simulink model "Modello_corretto_1dof"  (R2023b)
settings: Solver=VariableStepAuto  StartTime=0.0  StopTime=100  RelTol=1e-3
undefined symbols (not defined in the file or in its folder): param, tau_eq, Ts_slk, x0
settings Model: Creator=asus  LastModifiedBy=asus
settings OptimizationCC: ReuseModelBlockBuffer=off
settings DebuggingCC: SignalInfNanChecking=error

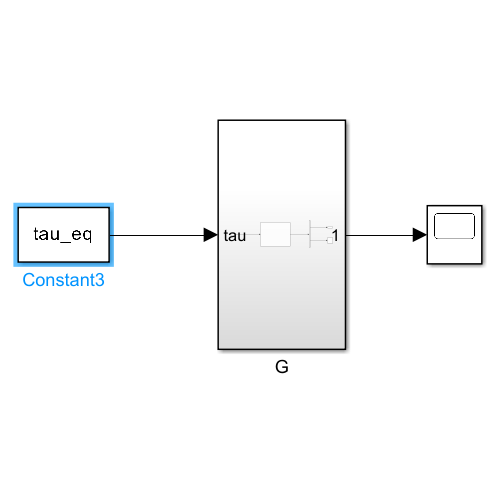
[thumbnail: Simulink's stored preview of the top-level diagram]
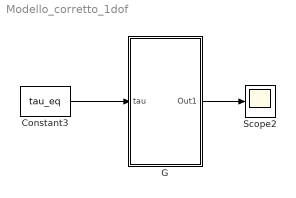
== system Modello_corretto_1dof ==
  Constant3 : Constant  Value=tau_eq  VectorParams1D=off  SampleTime=Ts_slk
  G : Subsystem
  Scope2 : Scope
  wires:
  Constant3/1 -> G/1("tau ")
  G/1(Out1) -> Scope2/1

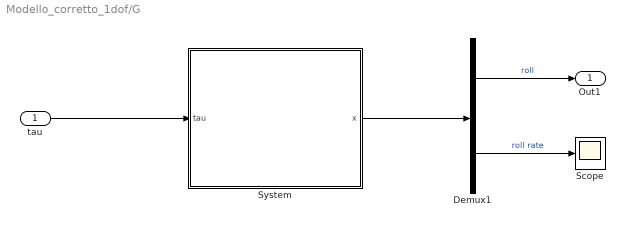
== system Modello_corretto_1dof/G ==
  "tau " : Inport
  Demux1 : Demux  Outputs=2
  Scope : Scope
  System : Subsystem
  Out1 : Outport
  wires:
  System/1(x) -> Demux1/1
  Demux1/1 -> Out1/1  "roll"
  Demux1/2 -> Scope/1  "roll rate"
  "tau "/1 -> System/1("tau ")

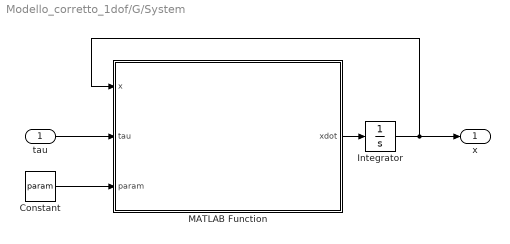
== system Modello_corretto_1dof/G/System ==
  "tau " : Inport
  Constant : Constant  Value=param
  Integrator : Integrator  InitialCondition=x0
  MATLAB Function : MATLAB Function  TreatAsAtomicUnit=on
  x : Outport
  wires:
  Integrator/1 -> MATLAB Function/1(x), x/1
  MATLAB Function/1(xdot) -> Integrator/1
  "tau "/1 -> MATLAB Function/2(tau)
  Constant/1 -> MATLAB Function/3(param)

== matlab function Modello_corretto_1dof/G/System/MATLAB Function ==
  data: x input; tau input; xdot output; param input
function xdot=quadcopter(x,tau,param)
% Inputs:
%           x       (model state)
%           tau     (torque)           
%           param   (model parameters)
%
% Outputs:  x_dot  (derivative of the state with respect to time)

% Parameters
g        =       9.81;           %  gravity acceleration (m/s^2)
Ixx      =       param(1,1);     %  moment of inertia 

% States
phi         =       x(1,1);      %  roll angle (rad)
phi_dot     =       x(2,1);      %  roll rate (rad/s)

cph         =       cos(phi);
sph         =       sin(phi);

% State space model
xdot        = zeros(2,1);
xdot(1,1)   = phi_dot;
xdot(2,1)   = tau/Ixx;
